simulink subsystem "pulse_extender"  (R2022b)
settings: Solver=VariableStepAuto  StartTime=0.0  StopTime=10.0  RelTol=1e-3
Description:
  | Copyright (c) 2023, Alexei Evsenin, evsenin@gmail.com
settings Model: Creator=evsenin  LastModifiedBy=evsenin
settings DebuggingCC: UnconnectedInputMsg=warning  UnconnectedOutputMsg=warning  UnconnectedLineMsg=warning
settings ModelReferenceCC: EnableRefExpFcnMdlSchedulingChecks=on
settings RTWCC: DLArmComputeVersion=19.05

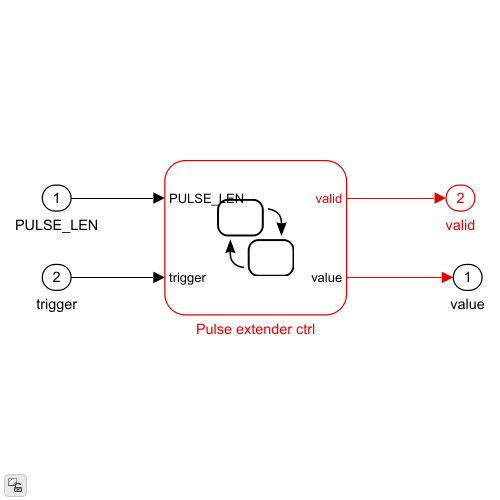
[thumbnail: Simulink's stored preview of the top-level diagram]
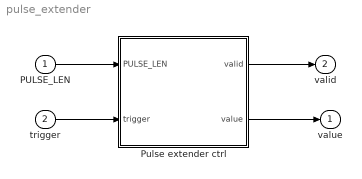
== system pulse_extender ==
  PULSE_LEN : Inport  OutDataTypeStr=uint16  PortDimensions=1
  trigger : Inport  Port=2  OutDataTypeStr=boolean  PortDimensions=1
  Pulse extender ctrl : Stateflow chart  TreatAsAtomicUnit=on
      settings: PortSchema="{\"entries\":[{\"content\":{\"sides\":[{\"content\":{\"connectorIds\":[\"Out1\",\"Out2\"]},\"type\":\"ConnectorPlacement.EquallySpacedRectSide\",\"uuid\":\"a7d5cd87-405a-43cf-8de2-83fd3c88d2fa\"},{\"content\":{\"connectorIds\":[\"In1\",\"In2\"],\"side\":\"RIGHT\"},\"type\":\"ConnectorPlacement.EquallySpacedRectSide\",\"uuid\":\"f771136f-2360-40d5-906d-70d6663b0e97\"},{\"content\":{\"connectorIds\":[],\"side\":\"TOP\"},\"type\":\"ConnectorPlacement.EquallySpacedRectSide\",\"uuid\":\"925d637f-1e07-494e-9726-80cfa838d753\"}]},\"type\":\"ConnectorPlacement.EquallySpacedConnector\",\"uuid\":\"2b760ece-89e2-4561-b843-8ad67cb6037f\"}],\"packageUris\":[\"http://schema.mathworks.com/mf0/Connector/R2020b\"],\"version\":\"1.0\"}"
  value : Outport  OutDataTypeStr=uint16  PortDimensions=1
  valid : Outport  Port=2  OutDataTypeStr=boolean  PortDimensions=1
  wires:
  trigger/1 -> Pulse extender ctrl/2(trigger)
  Pulse extender ctrl/2(value) -> value/1
  Pulse extender ctrl/1(valid) -> valid/1
  PULSE_LEN/1 -> Pulse extender ctrl/1(PULSE_LEN)

== stateflow chart pulse_extender/Pulse extender ctrl ==
  settings: executeAtInitialization=1
  state RESET
    valid = false;
    value = uint16(0);
  state VALID
    en:
    valid = true;
    value = 0;
    du:
    valid = true;
    value = value + 1;
    ex:
    valid = false;
  (default) -> RESET
  VALID -> RESET : [value == PULSE_LEN - 1]
  RESET -> VALID : [trigger]
  data: valid output boolean; PULSE_LEN input uint16; value output uint16; trigger input boolean
